simulink model "mmr_ground_beta_new"  (R2019a)
settings: Solver=VariableStepAuto  StartTime=0.0  StopTime=tc  RelTol=1e-1
values from neighbouring files (symbols this model uses):
  g = -9.81    [MMR.m]    (also in MMR_alfa0.m; MMR_alone.m; MMR_hop_zero.m = 9.81)
  k = 2000.0    (= 2000)    [MMR.m]    (also in MMR_alfa0.m = 22500; MMR_alone.m; MMR_hop_zero.m = 8515.125)
  L0 = sqrt(x0*x0 + y0*y0)    [MMR.m]    (also in MMR_alfa0.m; MMR_alone.m)
  Lcol = 0.70    (= 0.7)    [MMR.m]    (also in MMR_alone.m)
  Lhk = 0.28    [MMR.m]    (also in MMR_alfa0.m; MMR_alone.m; MMR_hop_zero.m)
  Lkf = 0.28    [MMR.m]    (also in MMR_alfa0.m; MMR_alone.m; MMR_hop_zero.m)
  M = 15    [MMR.m]    (also in MMR_alfa0.m; MMR_alone.m; MMR_hop_zero.m)
  m = 3    [MMR.m]    (also in MMR_alfa0.m; MMR_alone.m; MMR_hop_zero.m)
  vx0 = vxair( length(vxair) )    [MMR.m]    (also in MMR_alfa0.m = 0; MMR_alone.m)
  vxM0 = vxair( length(vxMair) )    [MMR.m]    (also in MMR_alfa0.m = 0; MMR_alone.m)
  vy0 = vyair( length(vyair) )    [MMR.m]    (also in MMR_alfa0.m = -0.7; MMR_alone.m; MMR_hop_zero.m = -0.613125)
  vyM0 = vyair( length(vyMair) )    [MMR.m]    (also in MMR_alfa0.m = -0.7; MMR_alone.m)
  x0 = Lkf * sin(alfa0 - beta0)    [MMR.m]    (also in MMR_alfa0.m = 0; MMR_alone.m)
  xM0 = x0 + Lhk*sin(alfa0)    [MMR.m]    (also in MMR_alfa0.m = 0; MMR_alone.m = x0 + Lhk*cos(alfa0))
  y0 = Lkf * cos(alfa0 - beta0)    [MMR.m]    (also in MMR_alfa0.m = 0.28; MMR_alone.m; MMR_hop_zero.m = 0.56)
  yM0 = y0 + Lhk * cos(alfa0)    [MMR.m]    (also in MMR_alfa0.m = 0.56; MMR_alone.m)
undefined symbols (not defined in the file or in its folder): magnitude
settings Model: Creator=Jesus  LastModifiedBy=Jesus
settings SolverCC: MaxConsecutiveMinStep=3

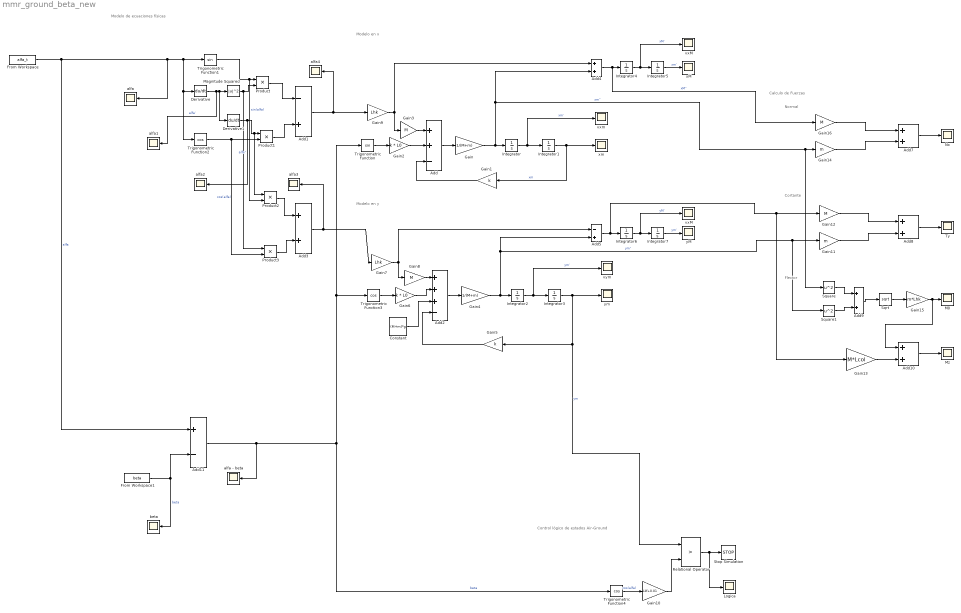
== system mmr_ground_beta_new ==
  note: Modelo de ecuaciones físicas
  note: Modelo en x
  note: Modelo en y
  note: Control lógico de estados Air-Ground
  note: Flector
  note: Normal
  note: Cortante
  note: Calculo de Fuerzas
  Add : Sum  Inputs=++-
  Add1 : Sum  Inputs=-+
  Add{3..4,7..10} (6 alike) : Sum
  Add11 : Sum  Inputs=+-
  Add2 : Sum  Inputs=+++-
  Add5 : Sum  Inputs=-+
  Constant : Constant  Value=(M+m)*g
  Derivative : Derivative  CoefficientInTFapproximation=1000
  Derivative1 : Derivative  CoefficientInTFapproximation=1000
  From Workspace : FromWorkspace  VariableName=alfa_t  SampleTime=0
  From Workspace1 : FromWorkspace  VariableName=beta  SampleTime=0
  Gain : Gain  Gain=1/(M+m)
  Gain1 : Gain  Gain=k
  Gain10 : Gain  Gain=Lkf+0.01
  Gain11 : Gain  Gain=m
  Gain{3,8,12,16} (4 alike) : Gain  Gain=M
  Gain13 : Gain  Gain=M*Lcol
  Gain14 : Gain  Gain=m
  Gain15 : Gain  Gain=m*Lhk
  Gain2 : Gain  Gain=k * L0
  Gain4 : Gain  Gain=1/(M+m)
  Gain5 : Gain  Gain=k
  Gain6 : Gain  Gain=k * L0
  Gain7 : Gain  Gain=Lhk
  Gain9 : Gain  Gain=Lhk
  Integrator : Integrator  InitialCondition=vx0
  Integrator1 : Integrator  InitialCondition=x0
  Integrator2 : Integrator  InitialCondition=vy0
  Integrator3 : Integrator  InitialCondition=y0
  Integrator4 : Integrator  InitialCondition=vxM0
  Integrator5 : Integrator  InitialCondition=xM0
  Integrator6 : Integrator  InitialCondition=vyM0
  Integrator7 : Integrator  InitialCondition=yM0
  Logica : Scope
  M0 : Scope
  Magnitude Squared : Math  Operator=magnitude^2  SaturateOnIntegerOverflow=on
  Mz : Scope
  Nx : Scope
  Product{,1..3} (4 alike) : Product
  Relational Operator : RelationalOperator  Operator=>  OutDataTypeStr=boolean  RndMeth=Simplest
  Sqrt : Sqrt  SaturateOnIntegerOverflow=on
  Square : Math  Operator=square  SaturateOnIntegerOverflow=on
  Square1 : Math  Operator=square  SaturateOnIntegerOverflow=on
  Stop Simulation : Stop
  Trigonometric Function : Trigonometry
  Trigonometric Function1 : Trigonometry
  Trigonometric Function2 : Trigonometry  Operator=cos
  Trigonometric Function3 : Trigonometry  Operator=cos
  Trigonometric Function4 : Trigonometry  Operator=cos
  Ty : Scope
  alfa{,1..4} (5 alike) : Scope
  alfa - beta : Scope
  beta : Scope
  vxM : Scope
  "vxM " : Scope
  vxm : Scope
  vym : Scope
  xM : Scope
  xm : Scope
  yM : Scope
  ym : Scope
  wires:
  Add/1 -> Gain/1
  Integrator/1 -> vxm/1, Integrator1/1  "xm'"
  Integrator1/1 -> Gain1/1, xm/1  "xm"
  Gain1/1 -> Add/3
  Gain2/1 -> Add/2
  Trigonometric Function/1 -> Gain2/1
  Add11/1 -> alfa - beta/1, Trigonometric Function4/1, Trigonometric Function/1, Trigonometric Function3/1  "beta"
  Trigonometric Function1/1 -> Product2/2, Product/1  "sin(alfa)"
  Derivative/1 -> alfa1/1, Derivative1/1, Magnitude Squared/1  "alfa'"
  Magnitude Squared/1 -> Product3/1, Product/2
  Derivative1/1 -> alfa2/1, Product1/1, Product2/1  "alfa''"
  Trigonometric Function2/1 -> Product3/2, Product1/2  "cos(alfa)"
  Product1/1 -> Add1/2
  Product/1 -> Add1/1
  Add1/1 -> Gain9/1, alfa4/1
  Gain3/1 -> Add/1
  Add2/1 -> Gain4/1
  Integrator2/1 -> vym/1, Integrator3/1  "ym'"
  Trigonometric Function3/1 -> Gain6/1
  Gain6/1 -> Add2/2
  Gain5/1 -> Add2/4
  Constant/1 -> Add2/3
  Product2/1 -> Add3/1
  Product3/1 -> Add3/2
  Add3/1 -> Gain7/1, alfa3/1
  Gain8/1 -> Add2/1
  Gain7/1 -> Add5/1, Gain8/1
  Gain9/1 -> Add4/1, Gain3/1
  Integrator4/1 -> "vxM "/1, Integrator5/1  "xM'"
  Integrator5/1 -> xM/1  "xm'"
  Integrator7/1 -> yM/1  "ym'"
  Integrator6/1 -> vxM/1, Integrator7/1  "yM'"
  Trigonometric Function4/1 -> Gain10/1  "cos(alfa)"
  Gain10/1 -> Relational Operator/2
  From Workspace/1 -> Add11/1, alfa/1, Trigonometric Function2/1, Derivative/1, Trigonometric Function1/1  "alfa"
  Relational Operator/1 -> Logica/1, Stop Simulation/1
  Integrator3/1 -> Relational Operator/1, Gain5/1, ym/1  "ym"
  Gain13/1 -> Add10/2
  Gain/1 -> Square/1, Gain14/1, Add4/2, Integrator/1  "xm''"
  Square/1 -> Add9/1
  Sqrt/1 -> Gain15/1
  Gain14/1 -> Add7/2
  Add9/1 -> Sqrt/1
  Add10/1 -> Mz/1
  Add8/1 -> Ty/1
  Gain12/1 -> Add8/1
  Gain4/1 -> Add5/2, Square1/1, Gain11/1, Integrator2/1  "ym''"
  Add4/1 -> Gain16/1, Integrator4/1  "xM''"
  Gain11/1 -> Add8/2
  Gain16/1 -> Add7/1
  Add7/1 -> Nx/1
  Add5/1 -> Gain12/1, Gain13/1, Integrator6/1
  Gain15/1 -> Add10/1, M0/1
  Square1/1 -> Add9/2
  From Workspace1/1 -> beta/1, Add11/2  "beta"
